simulink model "costas_pYll_gmsk"  (Simulink 7.1)
settings: Solver=VariableStepDiscrete  StartTime=0.0  StopTime=inf  RelTol=1e-3
libraries: dspsrcs4 x4, dsparch4 x3, simulink x2, commsynccomp2 x2, commchan3 x1
settings Model: Creator=Lekha1  LastModifiedBy=Lekha1

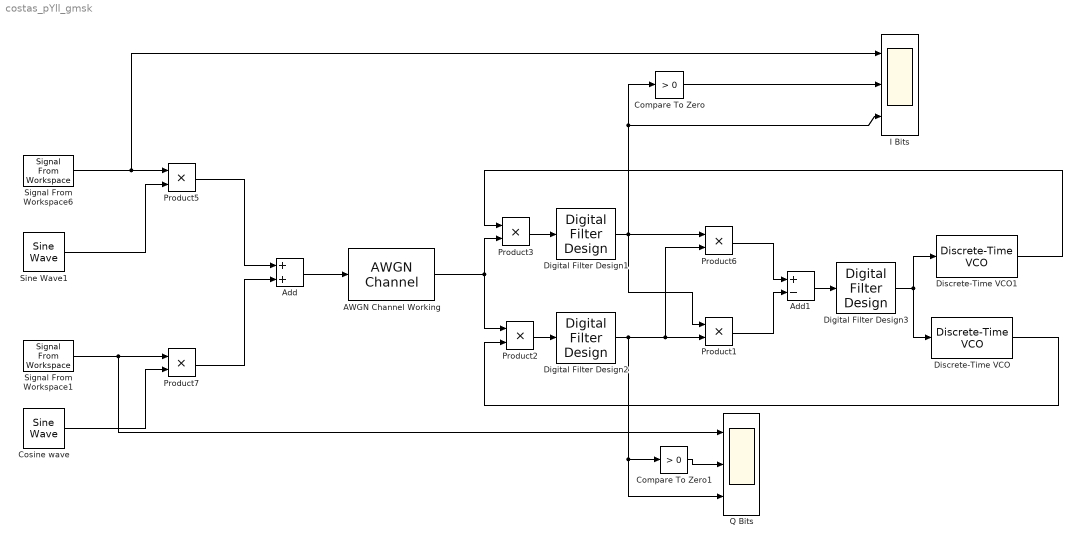
== system costas_pYll_gmsk ==
  AWGN Channel Working : commchan3/AWGN Channel  SystemSampleTime=-1  seed=67  noiseMode="Signal to noise ratio  (SNR)"  EbNodB=10  EsNodB=10  SNRdB=5  bitsPerSym=1  Ps=1  Tsym=1  variance=1
  Add : Sum  OutDataType=sfix(16)  OutScaling=2^-10
  Add1 : Sum  Inputs=+-  OutDataType=sfix(16)  OutScaling=2^-10
  Compare To Zero : simulink/Logic and Bit Operations/Compare To Zero  SystemSampleTime=-1  relop=>  LogicOutDataTypeMode=uint8  ZeroCross=off
  Compare To Zero1 : simulink/Logic and Bit Operations/Compare To Zero  SystemSampleTime=-1  relop=>  LogicOutDataTypeMode=uint8  ZeroCross=off
  Cosine wave : dspsrcs4/Sine Wave  Amplitude=1  Frequency=2e3  Phase=0  SampleMode=Discrete  OutComplex=Real  CompMethod=Trigonometric fcn  TableSize=Speed  SampleTime=1/(16*2e3)  SamplesPerFrame=1  dataType=double  wordLen=16  udDataType=sfix(16)  fracBitsMode=Best precision  numFracBits=15  ResetState=Restart at time zero
  Digital Filter Design1 : dsparch4/Digital Filter Design  SystemSampleTime=-1  mwdsp_browser_bugfix_var=off
  Digital Filter Design2 : dsparch4/Digital Filter Design  SystemSampleTime=-1  mwdsp_browser_bugfix_var=off
  Digital Filter Design3 : dsparch4/Digital Filter Design  SystemSampleTime=-1  mwdsp_browser_bugfix_var=off
  Discrete-Time VCO : commsynccomp2/Discrete-Time VCO  SystemSampleTime=-1  Ac=1  Fc=1e3  Kc=1e2  Ph=pi/2  ts=1/(16*1e3)
  Discrete-Time VCO1 : commsynccomp2/Discrete-Time VCO  SystemSampleTime=-1  Ac=1  Fc=1e3  Kc=1e2  Ph=0  ts=1/(16*1e3)
  I Bits : Scope  NumInputPorts=3
      settings: TimeRange=0.1799999999999997  YMin=0~0~-0.05  YMax=1~1~0.5
  Product{1..3,5..7} (6 alike) : Product  OutDataType=sfix(16)  OutScaling=2^0  RndMeth=Zero
  Q Bits : Scope  NumInputPorts=3
      settings: TimeRange=0.07199999999999995  YMin=0~0~-0.45  YMax=1~1~0.025
  Signal From Workspace1 : dspsrcs4/Signal From Workspace  SystemSampleTime=-1  X=Q_Signal  Ts=1/(640)  nsamps=1  OutputAfterFinalValue=Cyclic repetition  ignoreOrWarnInputAndFrameLengths=off
  Signal From Workspace6 : dspsrcs4/Signal From Workspace  SystemSampleTime=-1  X=I_Signal  Ts=1/(640)  nsamps=1  OutputAfterFinalValue=Cyclic repetition  ignoreOrWarnInputAndFrameLengths=off
  Sine Wave1 : dspsrcs4/Sine Wave  Amplitude=1  Frequency=2e3  Phase=pi/2  SampleMode=Discrete  OutComplex=Real  CompMethod=Trigonometric fcn  TableSize=Speed  SampleTime=1/(16*2e3)  SamplesPerFrame=1  dataType=double  wordLen=16  udDataType=sfix(16)  fracBitsMode=Best precision  numFracBits=15  ResetState=Restart at time zero
  wires:
  Compare To Zero/1 -> I Bits/2
  Digital Filter Design1/1 -> Product6/1, Product1/1, I Bits/3, Compare To Zero/1
  Digital Filter Design2/1 -> Product6/2, Product1/2, Q Bits/3, Compare To Zero1/1
  Digital Filter Design3/1 -> Discrete-Time VCO1/1, Discrete-Time VCO/1
  Product2/1 -> Digital Filter Design2/1
  Product3/1 -> Digital Filter Design1/1
  Discrete-Time VCO/1 -> Product2/2
  Compare To Zero1/1 -> Q Bits/2
  Product6/1 -> Add1/1
  Product1/1 -> Add1/2
  Add1/1 -> Digital Filter Design3/1
  Discrete-Time VCO1/1 -> Product3/1
  Signal From Workspace6/1 -> Product5/1, I Bits/1
  Signal From Workspace1/1 -> Product7/1, Q Bits/1
  Cosine wave/1 -> Product7/2
  Sine Wave1/1 -> Product5/2
  Add/1 -> AWGN Channel Working/1
  AWGN Channel Working/1 -> Product3/2, Product2/1
  Product7/1 -> Add/2
  Product5/1 -> Add/1
